simulink model "kalman_filter_linear"  (R2013a)
settings: Solver=ode4  StartTime=0.0  StopTime=20  FixedStep=0.01  MaxStep=0.01  RelTol=1e-3
libraries: dspmtrx3 x3
settings Model: Creator=CarlosMario  LastModifiedBy=Carlos Mario
settings DataIOCC: SignalLoggingSaveFormat=ModelDataLogs
settings OptimizationCC: InitFltsAndDblsToZero=on
settings DebuggingCC: SaveWithParameterizedLinksMsg=none  SignalResolutionControl=TryResolveAllWithWarning  MultiTaskDSMMsg=warning  MultiTaskCondExecSysMsg=none  FcnCallInpInsideContextMsg=UseLocalSettings  StrictBusMsg=None
settings RTWCC: SystemTargetFile=rtwin.tlc  TemplateMakefile=rtwin.tmf  Description=Real-Time Windows Target  ProcessScript=rtwin_make_rtw_hook  IncludeERTFirstTime=on
settings TargetCC: TargetFcnLib=ansi_tfl_tmw.mat  CodeReplacementLibrary=ANSI_C  IsPILTarget=off  ModelReferenceCompliant=off  CompOptLevelCompliant=off  EnableShiftOperators=on

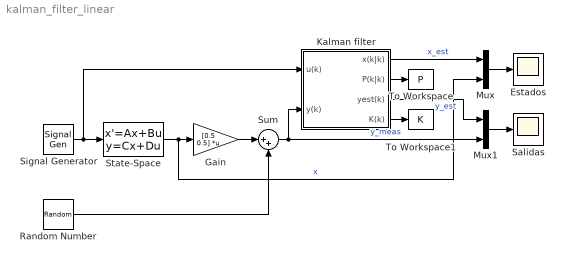
== system kalman_filter_linear ==
  Estados : Scope
      settings: ShowLegends=on
  Gain : Gain  Gain=[0.5 0.5]  Multiplication=Matrix(K*u)
  Kalman filter : Subsystem  mask(Linear Kalman Filter){Sd={[0.9801 -0.01485;0.0198 0.9999], [0.0198;0.0001987], [0.5 0.5]}, xuo={[0;0]          0}, PoQR={0.01*eye(2)          0.01*eye(2)           1}, T=0.01}
      mask prompts: Sd "{A,B,C} - Discrete-time system model"; xuo "{xo,uo} - Initial conditions"; PoQR "{Po,Q,R}"; T "T - Sample time"
      mask help:
      | Plant model:
      | x(k+1) = Ax(k) + Bu(k) + w(k)
      | y(k) = Cx(k) + v(k)
      |
      | E[x(0)-xo][x(0)-xo]' = Po      Ew(k)w'(k) = Q    Ev(k)v'(k) = R
      mask init:
      | A=Sd{1}; B=Sd{2}; C=Sd{3};
      | xo=xuo{1}; uo=xuo{2};
      | Po=PoQR{1}; Q=PoQR{2}; R=PoQR{3};
      mask Display:
      | disp('Kalman\nFilter')
      | port_label('input', 1, 'u')
      | port_label('input', 2, 'y')
      | port_label('output', 1, 'x')
      | port_label('output', 2, 'P')
      | port_label('output', 3, 'yest')
      | port_label('output', 4, 'K')
  Mux : Mux  Inputs=2
  Mux1 : Mux  Inputs=2
  Random Number : RandomNumber  Variance=0.1  SampleTime=0.01
  Salidas : Scope
      settings: ShowLegends=on  SaveName=ScopeData2
  Signal Generator : SignalGenerator  WaveForm=square  Frequency=0.1
  State-Space : StateSpace  A=[-2 -1.5;2 0]  B=[2;0]  C=[1 0;0 1]  D=[0;0]  X0=[0;0]
  Sum : Sum  Inputs=|++
  To Workspace : ToWorkspace  VariableName=P  SampleTime=-1
  To Workspace1 : ToWorkspace  VariableName=K  SampleTime=-1
  wires:
  Signal Generator/1 -> State-Space/1, Kalman filter/1(u(k))
  State-Space/1 -> Gain/1, Mux/2  "x"
  Gain/1 -> Sum/1
  Kalman filter/1(x(k|k)) -> Mux/1  "x_est"
  Mux/1 -> Estados/1
  Random Number/1 -> Sum/2
  Sum/1 -> Kalman filter/2(y(k)), Mux1/2  "y_meas"
  Mux1/1 -> Salidas/1
  Kalman filter/3(yest(k)) -> Mux1/1  "y_est"
  Kalman filter/2(P(k|k)) -> To Workspace/1
  Kalman filter/4(K(k)) -> To Workspace1/1

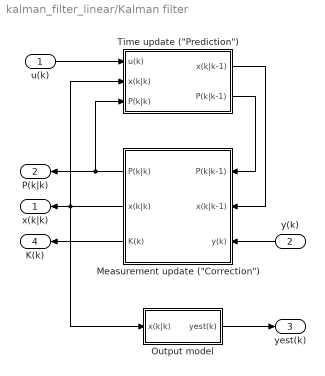
== system kalman_filter_linear/Kalman filter ==
  u(k) : Inport
  y(k) : Inport  Port=2
  "Measurement update (\"Correction\")" : Subsystem
  Output model : Subsystem
  "Time update (\"Prediction\")" : Subsystem
  x(k|k) : Outport
  P(k|k) : Outport  Port=2
  yest(k) : Outport  Port=3
  K(k) : Outport  Port=4
  wires:
  "Measurement update (\"Correction\")"/1(P(k|k)) -> "Time update (\"Prediction\")"/3(P(k|k)), P(k|k)/1
  u(k)/1 -> "Time update (\"Prediction\")"/1(u(k))
  y(k)/1 -> "Measurement update (\"Correction\")"/3(y(k))
  "Time update (\"Prediction\")"/2(P(k|k-1)) -> "Measurement update (\"Correction\")"/1(P(k|k-1))
  "Time update (\"Prediction\")"/1(x(k|k-1)) -> "Measurement update (\"Correction\")"/2(x(k|k-1))
  Output model/1(yest(k)) -> yest(k)/1
  "Measurement update (\"Correction\")"/2(x(k|k)) -> "Time update (\"Prediction\")"/2(x(k|k)), Output model/1(x(k|k)), x(k|k)/1
  "Measurement update (\"Correction\")"/3(K(k)) -> K(k)/1

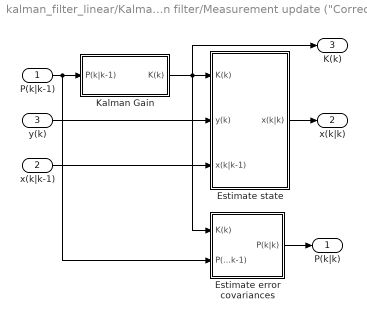
== system kalman_filter_linear/Kalman filter/Measurement update ("Correction") ==
  P(k|k-1) : Inport
  x(k|k-1) : Inport  Port=2
  y(k) : Inport  Port=3
  Estimate error covariances : Subsystem
  Estimate state : Subsystem
  Kalman Gain : Subsystem
  P(k|k) : Outport
  x(k|k) : Outport  Port=2
  K(k) : Outport  Port=3
  wires:
  P(k|k-1)/1 -> Kalman Gain/1(P(k|k-1)), Estimate error covariances/2(P(k|k-1))
  Kalman Gain/1(K(k)) -> Estimate state/1(K(k)), Estimate error covariances/1(K(k)), K(k)/1
  y(k)/1 -> Estimate state/2(y(k))
  Estimate state/1(x(k|k)) -> x(k|k)/1
  Estimate error covariances/1(P(k|k)) -> P(k|k)/1
  x(k|k-1)/1 -> Estimate state/3(x(k|k-1))

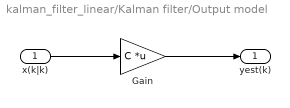
== system kalman_filter_linear/Kalman filter/Output model ==
  x(k|k) : Inport
  Gain : Gain  Gain=C  Multiplication=Matrix(K*u)  SampleTime=T
  yest(k) : Outport
  wires:
  x(k|k)/1 -> Gain/1
  Gain/1 -> yest(k)/1

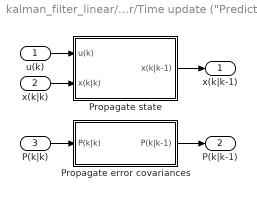
== system kalman_filter_linear/Kalman filter/Time update ("Prediction") ==
  u(k) : Inport
  x(k|k) : Inport  Port=2
  P(k|k) : Inport  Port=3
  Propagate error covariances : Subsystem
  Propagate state : Subsystem
  x(k|k-1) : Outport
  P(k|k-1) : Outport  Port=2
  wires:
  u(k)/1 -> Propagate state/1(u(k))
  Propagate state/1(x(k|k-1)) -> x(k|k-1)/1
  x(k|k)/1 -> Propagate state/2(x(k|k))
  P(k|k)/1 -> Propagate error covariances/1(P(k|k))
  Propagate error covariances/1(P(k|k-1)) -> P(k|k-1)/1

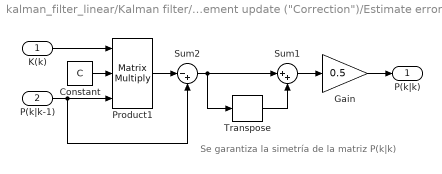
== system kalman_filter_linear/Kalman filter/Measurement update ("Correction")/Estimate error covariances ==
  note: Se garantiza la simetría
      | de la matriz P(k|k)
  K(k) : Inport
  P(k|k-1) : Inport  Port=2
  Constant : Constant  Value=C  VectorParams1D=off  SampleTime=T
  Gain : Gain  Gain=0.5  SampleTime=T
  Product1 : Product  Inputs=3  Multiplication=Matrix(*)  SampleTime=T  RndMeth=Zero
  Sum1 : Sum  Inputs=|++
  Sum2 : Sum  Inputs=|-+
  Transpose : dspmtrx3/Transpose  Hermitian=off  overflowFlag=on
  P(k|k) : Outport
  wires:
  Constant/1 -> Product1/2
  Product1/1 -> Sum2/1
  K(k)/1 -> Product1/1
  P(k|k-1)/1 -> Sum2/2, Product1/3
  Gain/1 -> P(k|k)/1
  Sum2/1 -> Sum1/1, Transpose/1
  Transpose/1 -> Sum1/2
  Sum1/1 -> Gain/1

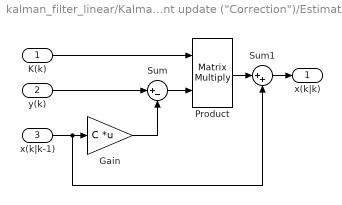
== system kalman_filter_linear/Kalman filter/Measurement update ("Correction")/Estimate state ==
  K(k) : Inport
  y(k) : Inport  Port=2
  x(k|k-1) : Inport  Port=3
  Gain : Gain  Gain=C  Multiplication=Matrix(K*u)  SampleTime=T
  Product : Product  Multiplication=Matrix(*)  SampleTime=T  RndMeth=Zero
  Sum : Sum  Inputs=|+-
  Sum1 : Sum  Inputs=|++
  x(k|k) : Outport
  wires:
  x(k|k-1)/1 -> Gain/1, Sum1/2
  Gain/1 -> Sum/2
  Sum/1 -> Product/2
  Product/1 -> Sum1/1
  K(k)/1 -> Product/1
  Sum1/1 -> x(k|k)/1
  y(k)/1 -> Sum/1

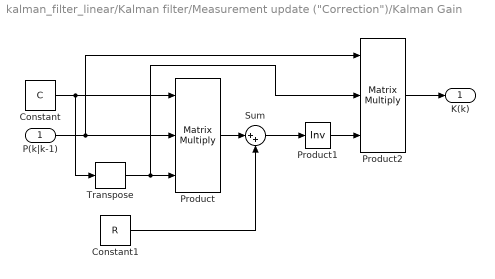
== system kalman_filter_linear/Kalman filter/Measurement update ("Correction")/Kalman Gain ==
  P(k|k-1) : Inport
  Constant : Constant  Value=C  VectorParams1D=off  SampleTime=T
  Constant1 : Constant  Value=R  SampleTime=T
  Product : Product  Inputs=3  Multiplication=Matrix(*)  SampleTime=T  RndMeth=Zero
  Product1 : Product  Inputs=/  Multiplication=Matrix(*)  SampleTime=T  RndMeth=Zero
  Product2 : Product  Inputs=3  Multiplication=Matrix(*)  SampleTime=T  RndMeth=Zero
  Sum : Sum  Inputs=|++
  Transpose : dspmtrx3/Transpose  Hermitian=off  overflowFlag=on
  K(k) : Outport
  wires:
  Constant/1 -> Product/1, Transpose/1
  P(k|k-1)/1 -> Product/2, Product2/1
  Transpose/1 -> Product/3, Product2/2
  Product/1 -> Sum/1
  Constant1/1 -> Sum/2
  Sum/1 -> Product1/1
  Product1/1 -> Product2/3
  Product2/1 -> K(k)/1

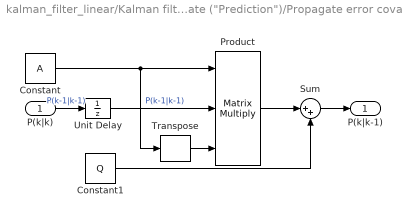
== system kalman_filter_linear/Kalman filter/Time update ("Prediction")/Propagate error covariances ==
  P(k|k) : Inport
  Constant : Constant  Value=A  SampleTime=T
  Constant1 : Constant  Value=Q  SampleTime=T
  Product : Product  Inputs=3  Multiplication=Matrix(*)  SampleTime=T  RndMeth=Zero
  Sum : Sum  Inputs=|++
  Transpose : dspmtrx3/Transpose  Hermitian=off  overflowFlag=on
  Unit Delay : UnitDelay  InitialCondition=Po  SampleTime=T
  P(k|k-1) : Outport
  wires:
  P(k|k)/1 -> Unit Delay/1  "P(k-1|k-1)"
  Constant/1 -> Product/1, Transpose/1
  Transpose/1 -> Product/3
  Product/1 -> Sum/1
  Constant1/1 -> Sum/2
  Sum/1 -> P(k|k-1)/1
  Unit Delay/1 -> Product/2  "P(k-1|k-1)"

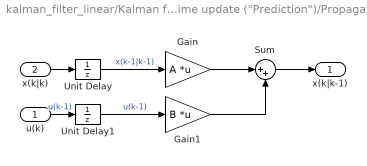
== system kalman_filter_linear/Kalman filter/Time update ("Prediction")/Propagate state ==
  u(k) : Inport
  x(k|k) : Inport  Port=2
  Gain : Gain  Gain=A  Multiplication=Matrix(K*u)  SampleTime=T
  Gain1 : Gain  Gain=B  Multiplication=Matrix(K*u)  SampleTime=T
  Sum : Sum  Inputs=|++
  Unit Delay : UnitDelay  InitialCondition=xo  SampleTime=T
  Unit Delay1 : UnitDelay  InitialCondition=uo  SampleTime=T
  x(k|k-1) : Outport
  wires:
  Unit Delay/1 -> Gain/1  "x(k-1|k-1)"
  x(k|k)/1 -> Unit Delay/1
  u(k)/1 -> Unit Delay1/1  "u(k-1)"
  Gain/1 -> Sum/1
  Gain1/1 -> Sum/2
  Sum/1 -> x(k|k-1)/1
  Unit Delay1/1 -> Gain1/1  "u(k-1)"
